simulink model "PID_controller_model"  (R2019a)
settings: Solver=VariableStepAuto  StartTime=0.0  StopTime=10.0  RelTol=1e-3
settings Model: Creator=賽維涅什  LastModifiedBy=賽維涅什

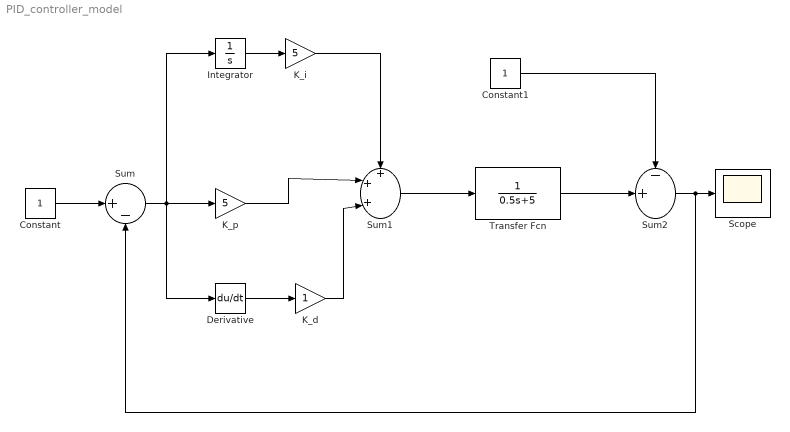
== system PID_controller_model ==
  Constant : Constant
  Constant1 : Constant
  Derivative : Derivative
  Integrator : Integrator
  K_d : Gain
  K_i : Gain  Gain=5
  K_p : Gain  Gain=5
  Scope : Scope
  Sum : Sum  Inputs=|+-
  Sum1 : Sum  Inputs=+++|
  Sum2 : Sum  Inputs=-+|
  Transfer Fcn : TransferFcn  Denominator=[0.5 5]
  wires:
  Constant/1 -> Sum/1
  Transfer Fcn/1 -> Sum2/2
  Sum/1 -> Derivative/1, Integrator/1, K_p/1
  Sum1/1 -> Transfer Fcn/1
  K_p/1 -> Sum1/2
  Integrator/1 -> K_i/1
  K_i/1 -> Sum1/1
  Derivative/1 -> K_d/1
  K_d/1 -> Sum1/3
  Constant1/1 -> Sum2/1
  Sum2/1 -> Scope/1, Sum/2
